simulink model "RFCcliTX_noExt"  (Simulink 7.4)
settings: Solver=FixedStepDiscrete  SolverMode=SingleTasking  StartTime=0.0  StopTime=inf  FixedStep=0.1  RelTol=1e-3
settings Model: Creator=fwornle  LastModifiedBy=fw  ExtModeTrigDuration=500
settings ConfigSet: Description=rtmc9s12target_R2008a
settings DataIOCC: SignalLoggingName=sigsOut
settings OptimizationCC: BooleanDataType=off  InitFltsAndDblsToZero=on
settings DebuggingCC: SaveWithParameterizedLinksMsg=none  SignalResolutionControl=TryResolveAllWithWarning  SolverPrmCheckMsg=none  MultiTaskDSMMsg=warning  MultiTaskCondExecSysMsg=none  StrictBusMsg=None
settings HardwareCC: ProdBitPerInt=16  ProdEndianess=BigEndian  ProdWordSize=16  ProdHWDeviceType=Motorola HC12  TargetHWDeviceType=32-bit Generic  ProdEqTarget=off
settings RTWCC: GenerateMakefile=off  TemplateMakefile=grt_msvc.tmf  Description="Visual C/C++ Project Makefile only for the \"grt\" target"  ProcessScript=grt_make_rtw_hook  IncludeERTFirstTime=on
settings GRTTargetCC: TargetFcnLib=ansi_tfl_tmw.mat

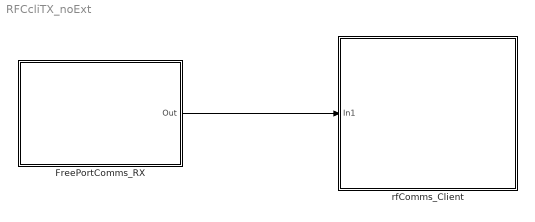
== system RFCcliTX_noExt ==
  FreePortComms_RX : Subsystem  Tag=mcTarget_freePortCommsRX  mask{sampletime=0.1, port=SCI0, baudrate=115200, channel=0, buf_size=5, data_type=UINT8, format=off, outformat=on}
      mask prompts: sampletime "Sample time"; port "Communication port"; channel "Channel number"; buf_size "Number of elements"; data_type "Data Type"; format "Block receives raw data"; outformat "Block output is double"
      mask init:
      | [buf_sizestr, portNamestr, baudratestr, channelstr, data_type_str, sampletime_str] = mbc_freeportrxd(sampletime, port, baudrate, channel, buf_size, data_type, format, outformat);
      mask Help: web('freePortComms_rxd.html');
      mask StyleString: edit,popup(SCI0|SCI1|COM1|COM2|COM3|COM4),popup(300|600|1200|2400|4800|9600|19200|38400|57600|115200),edit,edit,popup(SINGLE|INT8|UINT8|INT16|UINT16|INT32|UINT32|BOOLEAN),checkbox,checkbox
      mask Display: fprintf('Receive %s element(s)\nComm port: %s\nBaudrate: %s bps\nChannel: %s\nData type: %s\n Sample rate: %s', buf_sizestr, portNamestr, baudratestr, channelstr, data_type_str, sampletime_str)
  rfComms_Client : Subsystem  Tag=mcTarget_rfCommsCli  mask{sampletime=0.1, RXTXmode=Transmission (TX), RFchannel=12, clientNum=1, serverAddress=0xe7e7e7e7, clientAddress=0xc2c2c2c2, channel=0, buf_size=5, data_type=UINT8, format=on, outformat=on}
      mask prompts: sampletime "Sample time"; RXTXmode "Communication mode (TX, RX)"; RFchannel "RF channel number (0 - 127)"; clientNum "Client number"; serverAddress "Server address (4 bytes, hexadecimal notation, e.g. 0xe7e7e7e7)"; clientAddress "Client address (4 bytes, hexadecimal notation, e.g.: 0xc2c2c2c2)"; channel "User channel number (0 - 9)"; buf_size "Number of elements to be sent/received"; data_type "Data Type"; format "Block sends/receives raw data"; outformat "Block output is 'double'"
      mask init:
      | [buf_sizestr, RXTXmodestr, RFchannelstr, clientstr, serverAddressstr, clientAddressstr, channelstr, data_type_str, sampletime_str] = mbc_rfComms_client(sampletime, RXTXmode, RFchannel, clientNum, serverAddress, clientAddress, channel, buf_size, data_type, format, outformat);
      mask Help: web('rfComms_client.html');
      mask StyleString: edit,popup(Reception (RX)|Transmission (TX)),edit,popup(1|2|3|4|5),edit,edit,edit,edit,popup(SINGLE|INT8|UINT8|INT16|UINT16|INT32|UINT32|BOOLEAN),checkbox,checkbox
      mask Display: fprintf('RF mode: %s\nRF channel: %s\nClient: %s\nServer address: %s\nClient address: %s\nUser channel: %s\nElements: %s\nData type: %s\n Sample rate: %s', RXTXmodestr, RFchannelstr, clientstr, serverAddressstr, clientAddressstr, channelstr, buf_sizestr, data_type_str, sampletime_str)
  wires:
  FreePortComms_RX/1(Out) -> rfComms_Client/1(In1)

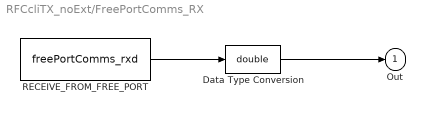
== system RFCcliTX_noExt/FreePortComms_RX ==
  Data Type Conversion : DataTypeConversion  OutDataTypeMode=double  OutDataType=sfix(16)  OutScaling=2^0  OutDataTypeStr=double  SaturateOnIntegerOverflow=on  RndMeth=Zero
  RECEIVE_FROM_FREE_PORT : S-Function  Tag=mcTarget_freePortCommsRX  FunctionName=freePortComms_rxd  Parameters=sampletime, channel, buf_size, data_type, port, baudrate, format  EnableBusSupport=off
  Out : Outport  OutDataType=sfix(16)  OutScaling=2^0
  wires:
  RECEIVE_FROM_FREE_PORT/1 -> Data Type Conversion/1
  Data Type Conversion/1 -> Out/1

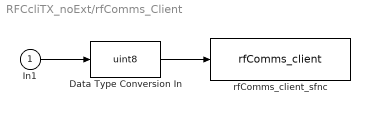
== system RFCcliTX_noExt/rfComms_Client ==
  In1 : Inport
  Data Type Conversion In : DataTypeConversion  OutDataTypeMode=uint8  OutDataTypeStr=uint8  SaturateOnIntegerOverflow=on  RndMeth=Zero
  rfComms_client_sfnc : S-Function  Tag=mcTarget_rfCommsCli  FunctionName=rfComms_client  Parameters=sampletime, RXTXmode, channel, buf_size, data_type  EnableBusSupport=off
  wires:
  Data Type Conversion In/1 -> rfComms_client_sfnc/1
  In1/1 -> Data Type Conversion In/1
